simulink model "rlAutoParkingValet"  (R2023a)
settings: Solver=VariableStepAuto  StartTime=0.0  StopTime=inf  RelTol=1e-3  AbsTol=1e-4
InitFcn:
  | setOccupied(map,1:64);
  | if doTraining == 0
  |     % set free spot
  |     setFree(map, freeSpotIdx);
  | else
  |     % free spot #7
  |     setFree(map,7);
  | end
undefined symbols (not defined in the file): doTraining, egoInitialPose, egoTargetPose, freeSpotIdx, lidarTol, map, maxLidarDist, numSensors, pTracking, speedMax, steerMax, terrTol, Tf, trainXBounds, trainYBounds, Ts, xBounds, Xref, xyerrTol, yBounds
libraries: mpclib x2, rllib x1
settings Model: PacingRate=0.089000  Creator=The MathWorks, Inc.  LastModifiedBy=Haykal
settings SolverCC: AutoScaleAbsTol=off  AlgebraicLoopSolver=TrustRegion  MinimalZcImpactIntegration=on
settings DebuggingCC: UnconnectedInputMsg=warning  UnconnectedOutputMsg=warning  UnconnectedLineMsg=warning
settings ModelReferenceCC: EnableRefExpFcnMdlSchedulingChecks=on
settings RTWCC: DLArmComputeVersion=19.05

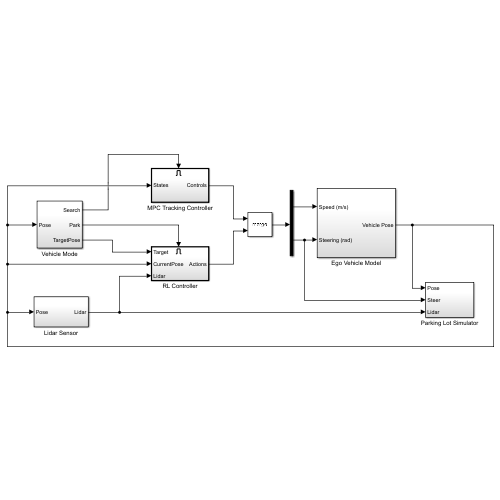
[thumbnail: Simulink's stored preview of the top-level diagram]
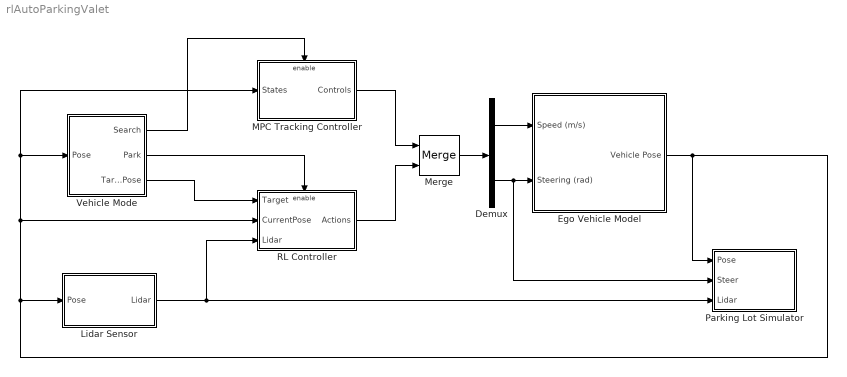
== system rlAutoParkingValet ==
  Demux : Demux  Outputs=2
  Ego Vehicle Model : Subsystem
  Lidar Sensor : Subsystem
  MPC Tracking Controller : Subsystem
  Merge : Merge
  Parking Lot Simulator : Subsystem
  RL Controller : Subsystem
  Vehicle Mode : Subsystem
  wires:
  Demux/1 -> Ego Vehicle Model/1(Speed (m/s))
  Demux/2 -> Parking Lot Simulator/2(Steer), Ego Vehicle Model/2(Steering (rad))
  Merge/1 -> Demux/1
  RL Controller/1(Actions) -> Merge/2
  MPC Tracking Controller/1(Controls) -> Merge/1
  Vehicle Mode/3(TargetPose) -> RL Controller/1(Target)
  Ego Vehicle Model/1(Vehicle Pose) -> MPC Tracking Controller/1(States), Vehicle Mode/1(Pose), RL Controller/2(CurrentPose), Lidar Sensor/1(Pose), Parking Lot Simulator/1(Pose)
  Lidar Sensor/1(Lidar) -> RL Controller/3(Lidar), Parking Lot Simulator/3(Lidar)
  Vehicle Mode/2(Park) -> RL Controller/Enable
  Vehicle Mode/1(Search) -> MPC Tracking Controller/Enable

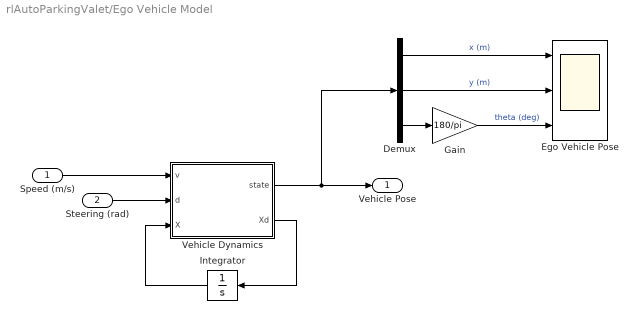
== system rlAutoParkingValet/Ego Vehicle Model ==
  Speed (m/s) : Inport
  Steering (rad) : Inport  Port=2
  Demux : Demux  Outputs=3
  Ego Vehicle Pose : Scope  NumInputPorts=3
  Gain : Gain  Gain=180/pi
  Integrator : Integrator  InitialCondition=egoInitialPose
  Vehicle Dynamics : Subsystem
  Vehicle Pose : Outport
  wires:
  Demux/3 -> Gain/1
  Demux/1 -> Ego Vehicle Pose/1  "x (m)"
  Demux/2 -> Ego Vehicle Pose/2  "y (m)"
  Speed (m/s)/1 -> Vehicle Dynamics/1(v)
  Steering (rad)/1 -> Vehicle Dynamics/2(d)
  Gain/1 -> Ego Vehicle Pose/3  "theta (deg)"
  Vehicle Dynamics/1(state) -> Demux/1, Vehicle Pose/1
  Vehicle Dynamics/2(Xd) -> Integrator/1
  Integrator/1 -> Vehicle Dynamics/3(X)

== system rlAutoParkingValet/Lidar Sensor ==
  Pose : Inport
  Demux : Demux  Outputs=3
  MATLAB System : MATLABSystem  System=LIDARSensor  MapObject=map  CarGeometry=map.VehicleDimensions  MaxDistance=maxLidarDist  SensorResolution=numSensors  ShowLIDARPlot=0  PlotLimits=[ xBounds yBounds ]
      mask Type: LIDARSensor
      mask Display:
      | disp('LIDARSensor');
      | port_label('input',1,'botx');
      | port_label('input',2,'boty');
      | port_label('input',3,'theta');
      | port_label('output',1,'d');
  Subsystem : Subsystem
  Lidar : Outport
  wires:
  Pose/1 -> Demux/1
  MATLAB System/1 -> Lidar/1
  Subsystem/1(centerX) -> MATLAB System/1
  Demux/2 -> Subsystem/2(currY)
  Demux/3 -> MATLAB System/3, Subsystem/3(theta)
  Demux/1 -> Subsystem/1(currX)
  Subsystem/2(centerY) -> MATLAB System/2

== system rlAutoParkingValet/MPC Tracking Controller ==
  States : Inport
  Enable : EnablePort  StatesWhenEnabling=reset
  Variant Subsystem : Subsystem  Variant=on  VariantControlMode=label  LabelModeActiveChoice=Choice_1  mask{choice=Adaptive MPC}
      mask init:
      | choice = get_param(gcb,'choice');
      | vssBlk = gcb;
      | oldVariant = get_param(gcb,'LabelModeActiveChoice');
      | if strcmp(choice,'Adaptive MPC')
      |     
      |     set_param(vssBlk, 'LabelModeActiveChoice', 'Choice_1');
      | else
      |     
      |     set_param(vssBlk, 'LabelModeActiveChoice', 'Choice_2');
      | end
      mask TypeOptions choice: Adaptive MPC | Nonlinear MPC
  Controls : Outport
  wires:
  States/1 -> Variant Subsystem/1(states)
  Variant Subsystem/1(controls) -> Controls/1

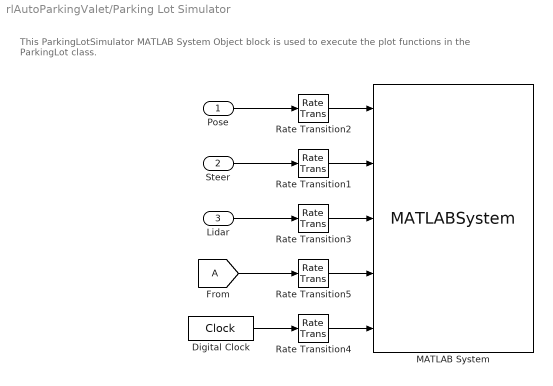
== system rlAutoParkingValet/Parking Lot Simulator ==
  note: This ParkingLotSimulator MATLAB System Object block is used to execute the plot functions in the ParkingLot class.
  Pose : Inport
  Steer : Inport  Port=2
  Lidar : Inport  Port=3
  Digital Clock : DigitalClock  SampleTime=Ts
  From : From  TagVisibility=global
  MATLAB System : MATLABSystem  System=ParkingLotSimulator  Visualization=1  MapObject=map  CameraDepth=cameraDepth  CameraViewAngle=cameraViewAngle  MaxLidarDistance=maxLidarDist  TrainingMode=doTraining
      mask Type: ParkingLotSimulator
      mask Display:
      | disp('ParkingLotSimulator');
      | port_label('input',1,'pose');
      | port_label('input',2,'steer');
      | port_label('input',3,'lidar');
      | port_label('input',4,'park');
      | port_label('input',5,'currentTime');
  Rate Transition{1..5} (5 alike) : RateTransition
  wires:
  Steer/1 -> Rate Transition1/1
  Pose/1 -> Rate Transition2/1
  Rate Transition1/1 -> MATLAB System/2
  Lidar/1 -> Rate Transition3/1
  From/1 -> Rate Transition5/1
  Digital Clock/1 -> Rate Transition4/1
  Rate Transition4/1 -> MATLAB System/5
  Rate Transition2/1 -> MATLAB System/1
  Rate Transition3/1 -> MATLAB System/3
  Rate Transition5/1 -> MATLAB System/4

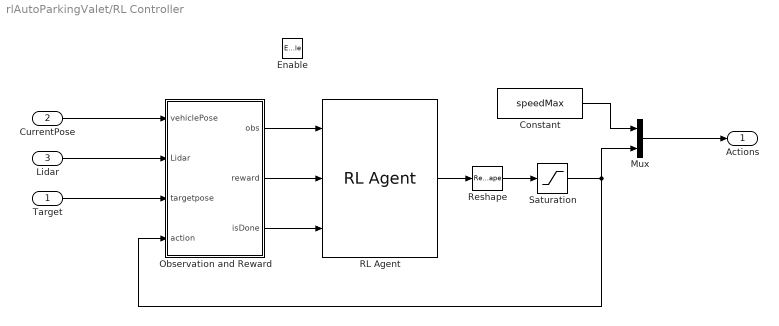
== system rlAutoParkingValet/RL Controller ==
  Target : Inport
  CurrentPose : Inport  Port=2
  Lidar : Inport  Port=3
  Enable : EnablePort  StatesWhenEnabling=reset
  Constant : Constant  Value=speedMax
  Mux : Mux  Inputs=2
  Observation and Reward : Subsystem
  RL Agent : rllib/RL Agent  Agent=agent  ExternalActionAsInput=off  ProvideLastAction=off  ProvideCumRwd=off  TreatAsDirectFeedthrough=on  UseStrictObservationDataTypes=off
  Reshape : Reshape
  Saturation : Saturate  UpperLimit=steerMax  LowerLimit=-steerMax
  Actions : Outport
  wires:
  Observation and Reward/1(obs) -> RL Agent/1
  Observation and Reward/2(reward) -> RL Agent/2
  Observation and Reward/3(isDone) -> RL Agent/3
  CurrentPose/1 -> Observation and Reward/1(vehiclePose)
  Target/1 -> Observation and Reward/3(targetpose)
  Lidar/1 -> Observation and Reward/2(Lidar)
  RL Agent/1 -> Reshape/1
  Saturation/1 -> Mux/2, Observation and Reward/4(action)
  Reshape/1 -> Saturation/1
  Constant/1 -> Mux/1
  Mux/1 -> Actions/1

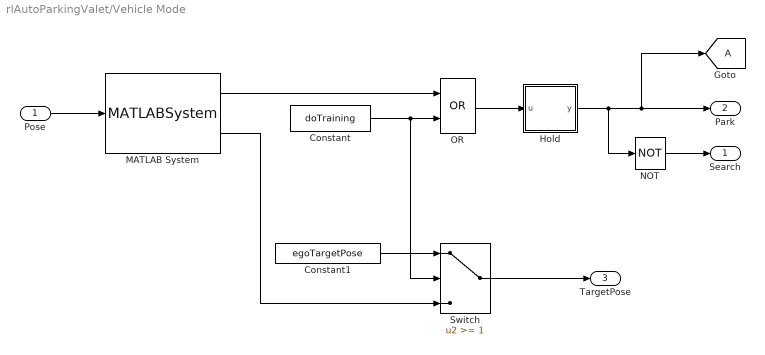
== system rlAutoParkingValet/Vehicle Mode ==
  Pose : Inport
  Constant : Constant  Value=doTraining
  Constant1 : Constant  Value=egoTargetPose
  Goto : Goto  TagVisibility=global
  Hold : Subsystem
  MATLAB System : MATLABSystem  System=Camera  MaxDepth=cameraDepth  MaxViewAngle=cameraViewAngle  MapObject=map
      mask Type: Camera
      mask Display:
      | disp('Camera');
      | port_label('input',1,'pose');
      | port_label('output',1,'found');
      | port_label('output',2,'goal');
  NOT : Logic  Operator=NOT  AllPortsSameDT=off  OutDataTypeStr=boolean
  OR : Logic  Operator=OR  AllPortsSameDT=off  OutDataTypeStr=boolean
  Switch : Switch  Threshold=1  SaturateOnIntegerOverflow=off  InputSameDT=off
  Search : Outport
  Park : Outport  Port=2
  TargetPose : Outport  Port=3
  wires:
  Pose/1 -> MATLAB System/1
  MATLAB System/1 -> OR/1
  OR/1 -> Hold/1(u)
  NOT/1 -> Search/1
  Hold/1(y) -> Goto/1, Park/1, NOT/1
  MATLAB System/2 -> Switch/3
  Constant1/1 -> Switch/1
  Switch/1 -> TargetPose/1
  Constant/1 -> Switch/2, OR/2

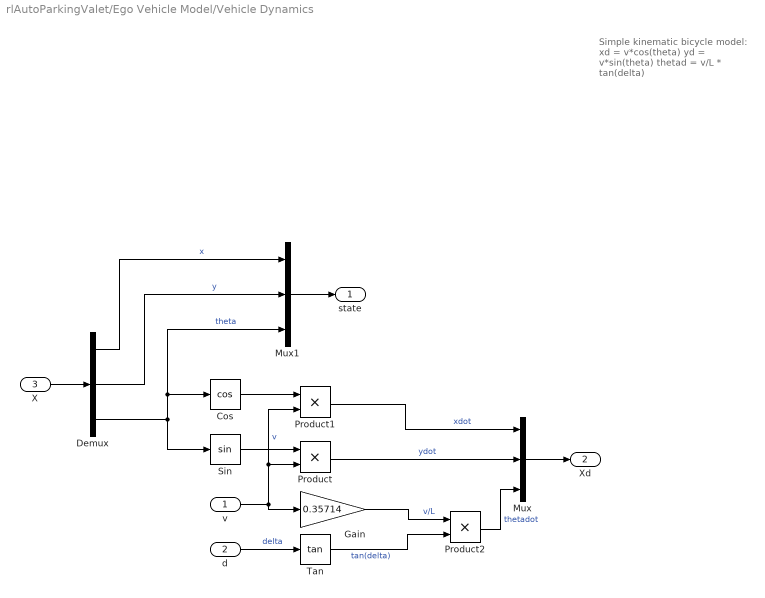
== system rlAutoParkingValet/Ego Vehicle Model/Vehicle Dynamics ==
  note: Simple kinematic bicycle model:
      |
      | xd = v*cos(theta)
      | yd = v*sin(theta)
      | thetad = v/L * tan(delta)
  v : Inport
  d : Inport  Port=2
  X : Inport  Port=3
  Cos : Trigonometry  Operator=cos
  Demux : Demux  Outputs=3
  Gain : Gain  Gain=0.35714
  Mux : Mux  Inputs=3
  Mux1 : Mux  Inputs=3
  Product : Product
  Product1 : Product
  Product2 : Product
  Sin : Trigonometry
  Tan : Trigonometry  Operator=tan
  state : Outport
  Xd : Outport  Port=2
  wires:
  Sin/1 -> Product/1
  Demux/3 -> Sin/1, Mux1/3, Cos/1  "theta"
  v/1 -> Gain/1, Product1/2, Product/2  "v"
  Cos/1 -> Product1/1
  d/1 -> Tan/1  "delta"
  Tan/1 -> Product2/2  "tan(delta)"
  Product/1 -> Mux/2  "ydot"
  Demux/1 -> Mux1/1  "x"
  Demux/2 -> Mux1/2  "y"
  Mux1/1 -> state/1
  Mux/1 -> Xd/1
  X/1 -> Demux/1
  Product1/1 -> Mux/1  "xdot"
  Product2/1 -> Mux/3  "thetadot"
  Gain/1 -> Product2/1  "v/L"

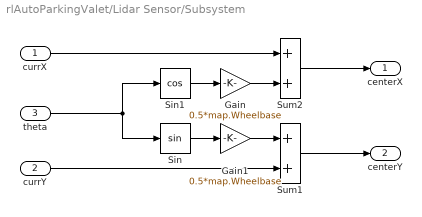
== system rlAutoParkingValet/Lidar Sensor/Subsystem ==
  currX : Inport
  currY : Inport  Port=2
  theta : Inport  Port=3
  Gain : Gain  Gain=0.5*map.Wheelbase
  Gain1 : Gain  Gain=0.5*map.Wheelbase
  Sin : Trigonometry
  Sin1 : Trigonometry  Operator=cos
  Sum1 : Sum
  Sum2 : Sum
  centerX : Outport
  centerY : Outport  Port=2
  wires:
  Sum1/1 -> centerY/1
  currY/1 -> Sum1/2
  theta/1 -> Sin/1, Sin1/1
  Sin/1 -> Gain1/1
  Sin1/1 -> Gain/1
  currX/1 -> Sum2/1
  Sum2/1 -> centerX/1
  Gain/1 -> Sum2/2
  Gain1/1 -> Sum1/1

== system rlAutoParkingValet/MPC Tracking Controller/Variant Subsystem ==
  note: 1) Add Subsystem or Model blocks as valid variant choices.
      | 2) You cannot connect blocks at this level. At simulation, connectivity is automatically
      | determined, based on the active variant and port name matching.
  states : Inport
  Adaptive MPC : Subsystem  VariantControl=Choice_1
  Nonlinear MPC : Subsystem  VariantControl=Choice_2
  controls : Outport

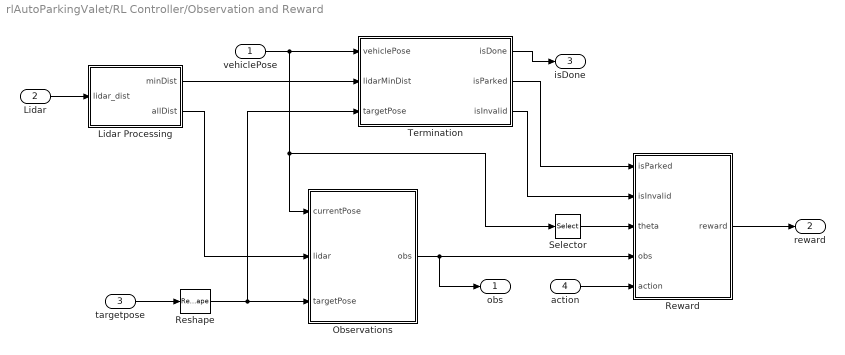
== system rlAutoParkingValet/RL Controller/Observation and Reward ==
  vehiclePose : Inport
  Lidar : Inport  Port=2
  targetpose : Inport  Port=3
  action : Inport  Port=4
  Lidar Processing : Subsystem
  Observations : Subsystem
  Reshape : Reshape
  Reward : Subsystem
  Selector : Selector  InputPortWidth=3  IndexOptions=Index vector (dialog)  Indices=3  OutputSizes=1
  Termination : Subsystem
  obs : Outport
  reward : Outport  Port=2
  isDone : Outport  Port=3
  wires:
  action/1 -> Reward/5(action)
  Reward/1(reward) -> reward/1
  targetpose/1 -> Reshape/1
  Lidar Processing/1(minDist) -> Termination/2(lidarMinDist)
  Lidar Processing/2(allDist) -> Observations/2(lidar)
  vehiclePose/1 -> Observations/1(currentPose), Selector/1, Termination/1(vehiclePose)
  Observations/1(obs) -> obs/1, Reward/4(obs)
  Lidar/1 -> Lidar Processing/1(lidar_dist)
  Selector/1 -> Reward/3(theta)
  Termination/2(isParked) -> Reward/1(isParked)
  Reshape/1 -> Termination/3(targetPose), Observations/3(targetPose)
  Termination/1(isDone) -> isDone/1
  Termination/3(isInvalid) -> Reward/2(isInvalid)

== system rlAutoParkingValet/Vehicle Mode/Hold ==
  u : Inport
  Add : Sum
  Data Type Conversion : DataTypeConversion  OutDataTypeStr=boolean  SaturateOnIntegerOverflow=off  RndMeth=Floor
  Data Type Conversion2 : DataTypeConversion  OutDataTypeStr=double  SaturateOnIntegerOverflow=off  RndMeth=Floor
  Memory : Memory
  Saturation : Saturate  UpperLimit=1  LowerLimit=0
  y : Outport
  wires:
  u/1 -> Data Type Conversion2/1
  Add/1 -> Saturation/1, Memory/1
  Memory/1 -> Add/2
  Saturation/1 -> Data Type Conversion/1
  Data Type Conversion/1 -> y/1
  Data Type Conversion2/1 -> Add/1

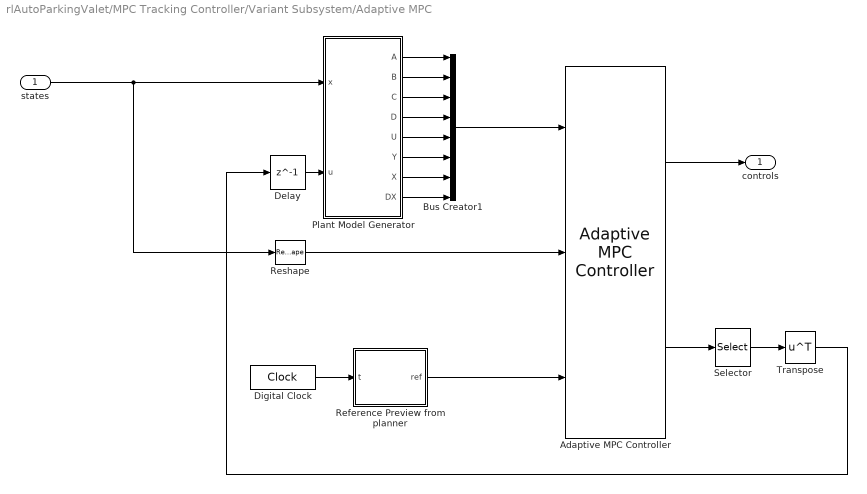
== system rlAutoParkingValet/MPC Tracking Controller/Variant Subsystem/Adaptive MPC ==
  states : Inport
  Adaptive MPC Controller : mpclib/Adaptive MPC Controller  SCDEnableBlockLinearizationSpecification=on  mpcobj=mpcobj  enable_value=0  updateMPCinCallerWorkspace=on  md_inport=off  mv_inport=off  uref_inport=off  return_cost=off  return_mvseq=on  return_qpstatus=off  return_xseq=off  return_state=off  return_ovseq=off  state_inport=on  isltv_plant=off  umin_inport=off  umax_inport=off  ymin_inport=off  ymax_inport=off  cc_inport=off  ywt_inport=off  uwt_inport=off  duwt_inport=off  rhoeps_inport=off  pm_inport=off  MaximumP=10  HorizonChoice=FixedHorizon  BlockDataType=double  SampleTimeInherited=off  switch_inport=off
  Bus Creator1 : BusCreator  Inputs=8
  Delay : Delay  DelayLength=1
  Digital Clock : DigitalClock  SampleTime=Ts
  Plant Model Generator : MATLAB Function  TreatAsAtomicUnit=on
  Reference Preview from planner : MATLAB Function  TreatAsAtomicUnit=on
  Reshape : Reshape  OutputDimensionality=Customize  OutputDimensions=[3,1]
  Selector : Selector  NumberOfDimensions=2  InputPortWidth=3  IndexOptions=Index vector (dialog),Select all  Indices=2,2  OutputSizes=1,1
  Transpose : Math  Operator=transpose  SignedPower=on
  controls : Outport
  wires:
  Adaptive MPC Controller/1 -> controls/1
  Selector/1 -> Transpose/1
  Delay/1 -> Plant Model Generator/2(u)
  Reshape/1 -> Adaptive MPC Controller/2
  Plant Model Generator/1(A) -> Bus Creator1/1
  Plant Model Generator/6(Y) -> Bus Creator1/6
  Transpose/1 -> Delay/1
  Plant Model Generator/3(C) -> Bus Creator1/3
  states/1 -> Reshape/1, Plant Model Generator/1(x)
  Plant Model Generator/8(DX) -> Bus Creator1/8
  Reference Preview from planner/1(ref) -> Adaptive MPC Controller/3
  Plant Model Generator/2(B) -> Bus Creator1/2
  Plant Model Generator/5(U) -> Bus Creator1/5
  Adaptive MPC Controller/2 -> Selector/1
  Plant Model Generator/4(D) -> Bus Creator1/4
  Plant Model Generator/7(X) -> Bus Creator1/7
  Digital Clock/1 -> Reference Preview from planner/1(t)
  Bus Creator1/1 -> Adaptive MPC Controller/1

== system rlAutoParkingValet/MPC Tracking Controller/Variant Subsystem/Nonlinear MPC ==
  states : Inport
  Delay : Delay  DelayLength=1
  Digital Clock : DigitalClock  SampleTime=Ts
  Nonlinear MPC Controller : mpclib/Nonlinear MPC Controller  SCDEnableBlockLinearizationSpecification=on  nlmpcobj=nlobjTracking  UseObjectTs=on  UseMEX=off  md_enabled=off  mvtarget_enabled=off  param_enabled=off  cost_enabled=off  mvseq_enabled=off  stateseq_enabled=off  ovseq_enabled=off  slack_enabled=off  status_enabled=off  ov_min=off  ov_max=off  mv_min=off  mv_max=off  mvrate_min=off  mvrate_max=off  state_min=off  state_max=off  ov_weight=off  mv_weight=off  mvrate_weight=off  ecr_weight=off  nlp_initialize=off
  Reference Preview from RRT : MATLAB Function  TreatAsAtomicUnit=on
  Reshape : Reshape  OutputDimensionality=Customize  OutputDimensions=[2,1]
  controls : Outport
  wires:
  Reference Preview from RRT/1(ref) -> Nonlinear MPC Controller/2
  Digital Clock/1 -> Reference Preview from RRT/1(t)
  Delay/1 -> Nonlinear MPC Controller/3
  states/1 -> Nonlinear MPC Controller/1
  Reshape/1 -> controls/1, Delay/1
  Nonlinear MPC Controller/1 -> Reshape/1

== system rlAutoParkingValet/RL Controller/Observation and Reward/Lidar Processing ==
  lidar_dist : Inport
  MATLAB Function : MATLAB Function  TreatAsAtomicUnit=on  mask{Res=numSensors, LW=map.VehicleDimensions}
      mask prompts: Res "Number of available measurements"; LW "Geometry of the car [L,W]"
      mask init:
      | res = Res;
      | L = LW(1);W = LW(2);
  MinMax : MinMax
  Sum : Sum  Inputs=|+-
  minDist : Outport
  allDist : Outport  Port=2
  wires:
  Sum/1 -> MinMax/1
  MATLAB Function/1(carDistances) -> Sum/2
  MinMax/1 -> minDist/1
  lidar_dist/1 -> Sum/1, allDist/1

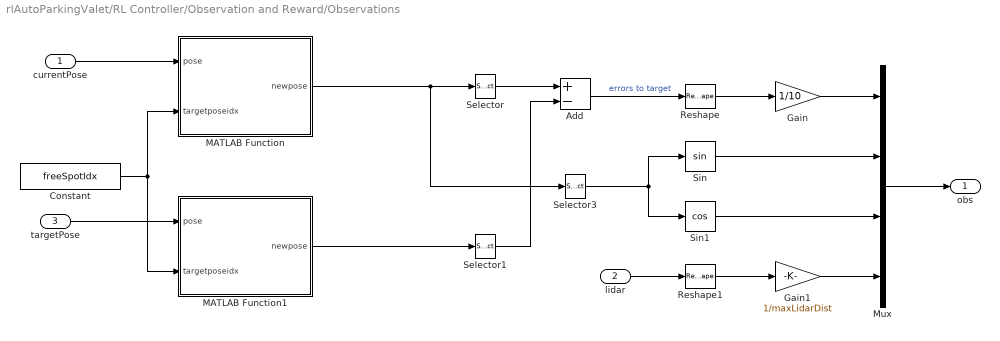
== system rlAutoParkingValet/RL Controller/Observation and Reward/Observations ==
  currentPose : Inport
  lidar : Inport  Port=2
  targetPose : Inport  Port=3
  Add : Sum  Inputs=+-
  Constant : Constant  Value=freeSpotIdx
  Gain : Gain  Gain=1/10
  Gain1 : Gain  Gain=1/maxLidarDist
  MATLAB Function : MATLAB Function  TreatAsAtomicUnit=on
  MATLAB Function1 : MATLAB Function  TreatAsAtomicUnit=on
  Mux : Mux
  Reshape : Reshape
  Reshape1 : Reshape
  Selector : Selector  InputPortWidth=3  IndexOptions=Index vector (dialog)  Indices=1:2  OutputSizes=1
  Selector1 : Selector  InputPortWidth=3  IndexOptions=Index vector (dialog)  Indices=1:2  OutputSizes=1
  Selector3 : Selector  InputPortWidth=3  IndexOptions=Index vector (dialog)  Indices=3  OutputSizes=1
  Sin : Trigonometry
  Sin1 : Trigonometry  Operator=cos
  obs : Outport
  wires:
  Reshape/1 -> Gain/1
  Add/1 -> Reshape/1  "errors to target"
  lidar/1 -> Reshape1/1
  Mux/1 -> obs/1
  Reshape1/1 -> Gain1/1
  Selector/1 -> Add/1
  Selector1/1 -> Add/2
  Sin/1 -> Mux/2
  Sin1/1 -> Mux/3
  Selector3/1 -> Sin/1, Sin1/1
  Gain/1 -> Mux/1
  Gain1/1 -> Mux/4
  Constant/1 -> MATLAB Function/2(targetposeidx), MATLAB Function1/2(targetposeidx)
  MATLAB Function/1(newpose) -> Selector3/1, Selector/1
  MATLAB Function1/1(newpose) -> Selector1/1
  currentPose/1 -> MATLAB Function/1(pose)
  targetPose/1 -> MATLAB Function1/1(pose)

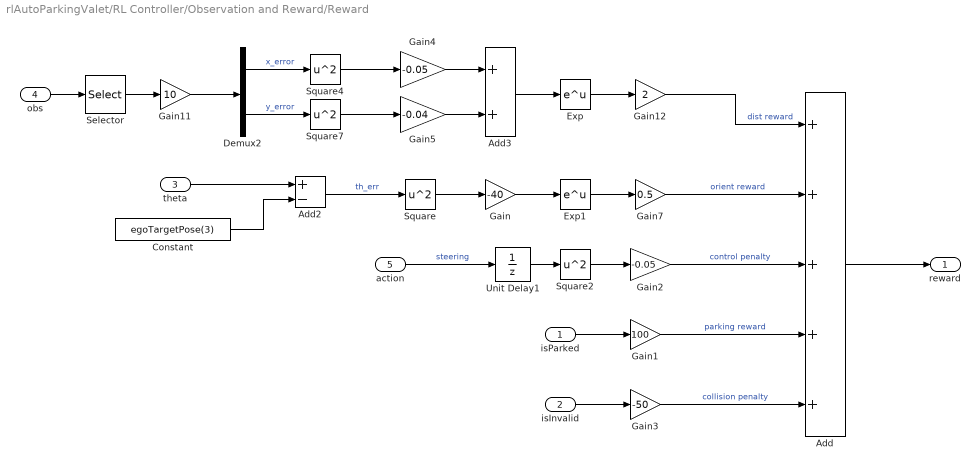
== system rlAutoParkingValet/RL Controller/Observation and Reward/Reward ==
  isParked : Inport
  isInvalid : Inport  Port=2
  theta : Inport  Port=3
  obs : Inport  Port=4
  action : Inport  Port=5
  Add : Sum  Inputs=+++++
  Add2 : Sum  Inputs=+-
  Add3 : Sum
  Constant : Constant  Value=egoTargetPose(3)
  Demux2 : Demux  Outputs=2
  Exp : Math
  Exp1 : Math
  Gain : Gain  Gain=-40
  Gain1 : Gain  Gain=100
  Gain11 : Gain  Gain=10
  Gain12 : Gain  Gain=2
  Gain2 : Gain  Gain=-0.05
  Gain3 : Gain  Gain=-50
  Gain4 : Gain  Gain=-0.05
  Gain5 : Gain  Gain=-0.04
  Gain7 : Gain  Gain=0.5
  Selector : Selector  InputPortWidth=numObservations  IndexOptions=Index vector (dialog)  Indices=1:2  OutputSizes=1
  Square{,2,4,7} (4 alike) : Math  Operator=square
  Unit Delay1 : UnitDelay  SampleTime=-1  HasFrameUpgradeWarning=on
  reward : Outport
  wires:
  action/1 -> Unit Delay1/1  "steering"
  Square2/1 -> Gain2/1
  Unit Delay1/1 -> Square2/1
  Add/1 -> reward/1
  Demux2/2 -> Square7/1  "y_error"
  Square7/1 -> Gain5/1
  Square4/1 -> Gain4/1
  Add3/1 -> Exp/1
  obs/1 -> Selector/1
  Demux2/1 -> Square4/1  "x_error"
  Gain4/1 -> Add3/1
  Gain5/1 -> Add3/2
  Exp/1 -> Gain12/1
  Selector/1 -> Gain11/1
  Add2/1 -> Square/1  "th_err"
  Square/1 -> Gain/1
  Gain/1 -> Exp1/1
  Constant/1 -> Add2/2
  theta/1 -> Add2/1
  Gain2/1 -> Add/3  "control penalty"
  Exp1/1 -> Gain7/1
  Gain12/1 -> Add/1  "dist reward"
  Gain7/1 -> Add/2  "orient reward"
  Gain11/1 -> Demux2/1
  isParked/1 -> Gain1/1
  Gain1/1 -> Add/4  "parking reward"
  isInvalid/1 -> Gain3/1
  Gain3/1 -> Add/5  "collision penalty"

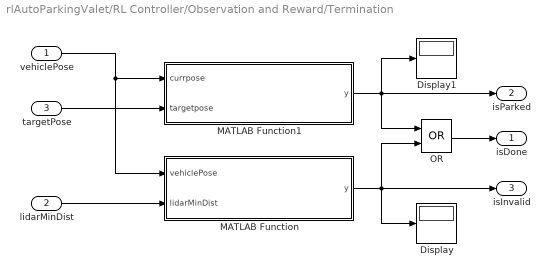
== system rlAutoParkingValet/RL Controller/Observation and Reward/Termination ==
  vehiclePose : Inport
  lidarMinDist : Inport  Port=2
  targetPose : Inport  Port=3
  Display : Display
  Display1 : Display
  MATLAB Function : MATLAB Function  TreatAsAtomicUnit=on
  MATLAB Function1 : MATLAB Function  TreatAsAtomicUnit=on
  OR : Logic  Operator=OR  AllPortsSameDT=off  OutDataTypeStr=boolean
  isDone : Outport
  isParked : Outport  Port=2
  isInvalid : Outport  Port=3
  wires:
  vehiclePose/1 -> MATLAB Function/1(vehiclePose), MATLAB Function1/1(currpose)
  lidarMinDist/1 -> MATLAB Function/2(lidarMinDist)
  OR/1 -> isDone/1
  targetPose/1 -> MATLAB Function1/2(targetpose)
  MATLAB Function1/1(y) -> Display1/1, isParked/1, OR/1
  MATLAB Function/1(y) -> OR/2, isInvalid/1, Display/1

== matlab function rlAutoParkingValet/RL Controller/Observation and Reward/Termination/MATLAB Function ==
  data: vehiclePose input; lidarMinDist input; y output; xBounds parameter; yBounds parameter; trainXBounds parameter; trainYBounds parameter; doTraining parameter; lidarTol parameter
function y = isOutOfBounds(vehiclePose, lidarMinDist, xBounds, yBounds, trainXBounds, trainYBounds, doTraining, lidarTol)

if doTraining
    xlims = trainXBounds;
    ylims = trainYBounds;
else
    xlims = xBounds;
    ylims = yBounds;
end

% get coordinates of four corners
xc = vehiclePose(1);
yc = vehiclePose(2);
t  = vehiclePose(3);

% Check if true positions are out of bounds
xOutOfBounds = xc <= xlims(1) || xc >= xlims(2);
yOutOfBounds = yc <= ylims(1) || yc >= ylims(2);

% check if lidar reading is less than threshold value
veryCloseToObstacle = lidarMinDist <= lidarTol;

goingInCircles = false;
if doTraining
    goingInCircles = t > 2*pi;
end

y = xOutOfBounds || yOutOfBounds || veryCloseToObstacle || goingInCircles;

== matlab function rlAutoParkingValet/RL Controller/Observation and Reward/Observations/MATLAB Function ==
  data: pose input; newpose output; targetposeidx input
function newpose = transformPose(pose,targetposeidx)

x = pose(1,:);
y = pose(2,:);
t = pose(3,:);

if targetposeidx > 14 && targetposeidx <= 22
    x =  pose(2);
    y = 100 - pose(1);
    t = pose(3) - pi/2;
elseif targetposeidx > 22 && targetposeidx <= 36
    x = 100 - pose(1);
    y = 60 - pose(2);
    t = pose(3) - pi;
elseif targetposeidx > 36 && targetposeidx <= 40
    x = 60 - pose(2);
    y = pose(1);
    t = pose(3) - 3*pi/2;
elseif targetposeidx > 40 && targetposeidx <= 52
    x = 100 - pose(1);
    y = 30 - pose(2);
    t = pi + pose(3);
elseif targetposeidx > 52 && targetposeidx <= 64
    x = pose(1);
    y = pose(2) - 28;
    t = pose(3);
end

newpose = [x y t]';

== matlab function rlAutoParkingValet/RL Controller/Observation and Reward/Lidar Processing/MATLAB Function ==
  data: carDistances output; W parameter; L parameter; res parameter
function carDistances = getDistances2CarBoundary(W,L,res)

angles = (0:(res-1))*2*pi/res;
carDistances = getCarSegmentLengths(L,W,angles);

== matlab function rlAutoParkingValet/MPC Tracking Controller/Variant Subsystem/Nonlinear MPC/Reference Preview from RRT ==
  data: t input; ref output; Ts parameter; Tf parameter; pTracking parameter; Xref parameter
function ref = fcn(t,Ts,Tf,pTracking,Xref)
Tend = Tf;
T = t+(1:pTracking)*Ts;
T = min(T,Tend);
time = Ts*(1:length(Xref));
ref = interp1(time,Xref,T);

== matlab function rlAutoParkingValet/RL Controller/Observation and Reward/Termination/MATLAB Function1 ==
  data: currpose input; y output; targetpose input; xyerrTol parameter; terrTol parameter
function y = isParked(currpose,targetpose, xyerrTol, terrTol)

x = currpose(1);
y = currpose(2);
t = currpose(3);
xg = targetpose(1);
yg = targetpose(2);
tg = targetpose(3);
xyerr = sqrt((x-xg)^2+(y-yg)^2);
terr = t-tg;
y = 0;
if xyerr < xyerrTol && abs(terr) < terrTol
    y = 1;
end

== matlab function rlAutoParkingValet/RL Controller/Observation and Reward/Observations/MATLAB Function1 ==
  data: pose input; newpose output; targetposeidx input
function newpose = transformPose(pose,targetposeidx)

x = pose(1,:);
y = pose(2,:);
t = pose(3,:);

if targetposeidx > 14 && targetposeidx <= 22
    x =  pose(2);
    y = 100 - pose(1);
    t = pose(3) - pi/2;
elseif targetposeidx > 22 && targetposeidx <= 36
    x = 100 - pose(1);
    y = 60 - pose(2);
    t = pose(3) - pi;
elseif targetposeidx > 36 && targetposeidx <= 40
    x = 60 - pose(2);
    y = pose(1);
    t = pose(3) - 3*pi/2;
elseif targetposeidx > 40 && targetposeidx <= 52
    x = 100 - pose(1);
    y = 30 - pose(2);
    t = pi + pose(3);
elseif targetposeidx > 52 && targetposeidx <= 64
    x = pose(1);
    y = pose(2) - 28;
    t = pose(3);
end

newpose = [x y t]';

== matlab function rlAutoParkingValet/MPC Tracking Controller/Variant Subsystem/Adaptive MPC/Plant Model Generator ==
  settings: updateMethod=DISCRETE  sampleTime=Ts
  data: x input size=[3,1]; u input size=[2,1]; A output; B output; C output; D output; U output size=[2,1]; Y output size=[3,1]; X output size=[3,1]; DX output size=[3,1]; Ts parameter
function [A,B,C,D,U,Y,X,DX] = fcn(x,u,Ts)

[A,B,C,D,U,Y,X,DX] = vehicleStateJacobianFcnDT(Ts,x,u);

== matlab function rlAutoParkingValet/MPC Tracking Controller/Variant Subsystem/Adaptive MPC/Reference Preview from planner ==
  data: t input; ref output; Ts parameter; Tf parameter; pTracking parameter; Xref parameter
function ref = fcn(t,Ts,Tf,pTracking,Xref)
Tend = Tf;
T = t+(1:pTracking)*Ts;
T = min(T,Tend);
time = Ts*(1:length(Xref*1.2));
ref = interp1(time,Xref,T);
